simulink model "HVAC_EX"  (Simulink 7.1)
settings: Solver=FixedStepDiscrete  StartTime=0.0  StopTime=40  FixedStep=1  RelTol=1e-3
undefined symbols (not defined in the file or in its folder): AR_A, AR_C, mix_A, mix_C
libraries: MPCMdlLib x21
settings Model: Creator=vichik  LastModifiedBy=vichik

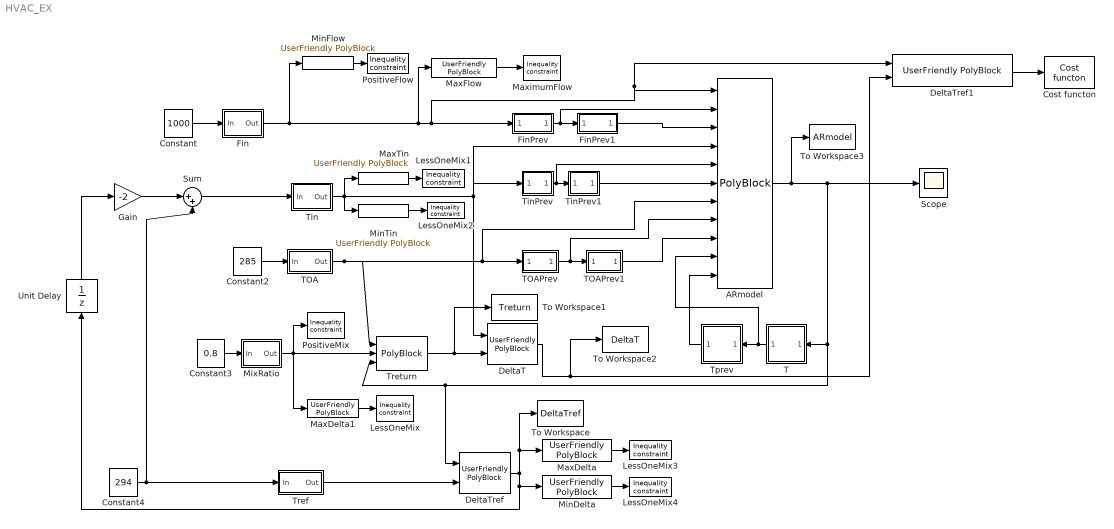
== system HVAC_EX ==
  ARmodel : MPCMdlLib/PolyBlock  Tag=PolyBlock  A=AR_A  C=AR_C
  Constant : Constant  Value=1000  OutDataType=sfix(16)  OutScaling=2^0
  Constant2 : Constant  Value=285  OutDataType=sfix(16)  OutScaling=2^0
  Constant3 : Constant  Value=0.8  OutDataType=sfix(16)  OutScaling=2^0
  Constant4 : Constant  Value=294  OutDataType=sfix(16)  OutScaling=2^0
  Cost functon : MPCMdlLib/Cost functon  Tag=OptCost
  DeltaT : MPCMdlLib/UserFriendly PolyBlock  Tag=PolyBlock  A="[1  0  ; 0 1 ]"  C="[1  -1]"  gA=[0 0]  gC=1
  DeltaTref : MPCMdlLib/UserFriendly PolyBlock  Tag=PolyBlock  A="[1  0  ; 0 1 ]"  C="[1  -1]"  gA=[0 0]  gC=1
  DeltaTref1 : MPCMdlLib/UserFriendly PolyBlock  Tag=PolyBlock  A="[2  0  ; 0 2 ]"  C=[0.00001 1]  gA=[0 0]  gC=1
  Fin : Subsystem  Tag=OptInput  AncestorBlock=MPCMdlLib/Input var  mask{step_ratio=1}
      mask prompts: step_ratio "Step ratio"
      mask Display: fprintf('Input')
  FinPrev : Subsystem  Tag=OptState  AncestorBlock=MPCMdlLib/state  mask{init_val=1000}
      mask prompts: init_val "Initial value"
      mask Display: fprintf('state')
  FinPrev1 : Subsystem  Tag=OptState  AncestorBlock=MPCMdlLib/state  mask{init_val=1000}
      mask prompts: init_val "Initial value"
      mask Display: fprintf('state')
  Gain : Gain  Gain=-2  ParameterDataType=sfix(16)  ParameterScaling=2^0  OutDataType=sfix(16)  OutScaling=2^0
  LessOneMix{,1..4} (5 alike) : MPCMdlLib/Inequality constraint  Tag=InequalBlock  CompareSign=> 0
  MaxDelta : MPCMdlLib/UserFriendly PolyBlock  Tag=PolyBlock  A="[0  ;1]"  C=[2 -1]  gA=[0 ]  gC=1
  MaxDelta1 : MPCMdlLib/UserFriendly PolyBlock  Tag=PolyBlock  A="[0  ;1]"  C=[1 -1]  gA=[0 ]  gC=1
  MaxFlow : MPCMdlLib/UserFriendly PolyBlock  Tag=PolyBlock  A="[0  ; 1]"  C=[4000 -1]  gA=[0 ]  gC=1
  MaxTin : MPCMdlLib/UserFriendly PolyBlock  Tag=PolyBlock  A="[0  ; 1]"  C=[310 -1]  gA=[0 ]  gC=1
  MaximumFlow : MPCMdlLib/Inequality constraint  Tag=InequalBlock  CompareSign=> 0
  MinDelta : MPCMdlLib/UserFriendly PolyBlock  Tag=PolyBlock  A="[1  ; 0]"  C=[1 2]  gA=[0 ]  gC=1
  MinFlow : MPCMdlLib/UserFriendly PolyBlock  Tag=PolyBlock  A="[1  ; 0]"  C=[1 -50]  gA=[0 ]  gC=1
  MinTin : MPCMdlLib/UserFriendly PolyBlock  Tag=PolyBlock  A="[1  ; 0]"  C=[1 -260]  gA=[0 ]  gC=1
  MixRatio : Subsystem  Tag=OptInput  AncestorBlock=MPCMdlLib/Input var  mask{step_ratio=1}
      mask prompts: step_ratio "Step ratio"
      mask Display: fprintf('Input')
  PositiveFlow : MPCMdlLib/Inequality constraint  Tag=InequalBlock  CompareSign=> 0
  PositiveMix : MPCMdlLib/Inequality constraint  Tag=InequalBlock  CompareSign=> 0
  Scope : Scope
      settings: TimeRange=10
  Sum : Sum  Inputs=|++  OutDataType=sfix(16)  OutScaling=2^0
  T : Subsystem  Tag=OptState  Orientation=left  AncestorBlock=MPCMdlLib/state  mask{init_val=293}
      mask prompts: init_val "Initial value"
      mask Display: fprintf('state')
  TOA : Subsystem  Tag=OptExternal  AncestorBlock=MPCMdlLib/External Var
      mask Display: fprintf('External')
  TOAPrev : Subsystem  Tag=OptState  AncestorBlock=MPCMdlLib/state  mask{init_val=285}
      mask prompts: init_val "Initial value"
      mask Display: fprintf('state')
  TOAPrev1 : Subsystem  Tag=OptState  AncestorBlock=MPCMdlLib/state  mask{init_val=285}
      mask prompts: init_val "Initial value"
      mask Display: fprintf('state')
  Tin : Subsystem  Tag=OptInput  AncestorBlock=MPCMdlLib/Input var  mask{step_ratio=1}
      mask prompts: step_ratio "Step ratio"
      mask Display: fprintf('Input')
  TinPrev : Subsystem  Tag=OptState  AncestorBlock=MPCMdlLib/state  mask{init_val=294}
      mask prompts: init_val "Initial value"
      mask Display: fprintf('state')
  TinPrev1 : Subsystem  Tag=OptState  AncestorBlock=MPCMdlLib/state  mask{init_val=294}
      mask prompts: init_val "Initial value"
      mask Display: fprintf('state')
  To Workspace : ToWorkspace  VariableName=DeltaTref  SampleTime=-1  SaveFormat=Structure
  To Workspace1 : ToWorkspace  VariableName=Treturn  SampleTime=-1  SaveFormat=Structure
  To Workspace2 : ToWorkspace  VariableName=DeltaT  SampleTime=-1  SaveFormat=Structure
  To Workspace3 : ToWorkspace  VariableName=ARmodel  SampleTime=-1  SaveFormat=Structure With Time
  Tprev : Subsystem  Tag=OptState  Orientation=left  AncestorBlock=MPCMdlLib/state  mask{init_val=293}
      mask prompts: init_val "Initial value"
      mask Display: fprintf('state')
  Tref : Subsystem  Tag=OptExternal  AncestorBlock=MPCMdlLib/External Var
      mask Display: fprintf('External')
  Treturn : MPCMdlLib/PolyBlock  Tag=PolyBlock  A=mix_A  C=mix_C
  Unit Delay : UnitDelay  Orientation=up  SampleTime=-1
  wires:
  Constant/1 -> Fin/1(In)
  Fin/1(Out) -> FinPrev/1(In1), ARmodel/1, DeltaTref1/1, MaxFlow/1, MinFlow/1
  Tin/1(Out) -> TinPrev/1(In1), DeltaT/1, ARmodel/4, MinTin/1, MaxTin/1
  FinPrev/1(Out1) -> FinPrev1/1(In1), ARmodel/2
  Constant2/1 -> TOA/1(In)
  TOA/1(Out) -> Treturn/1, TOAPrev/1(In1), ARmodel/7
  MaxFlow/1 -> MaximumFlow/1
  Constant3/1 -> MixRatio/1(In)
  MixRatio/1(Out) -> PositiveMix/1, MaxDelta1/1, Treturn/2
  MaxDelta1/1 -> LessOneMix/1
  MaxTin/1 -> LessOneMix1/1
  MinTin/1 -> LessOneMix2/1
  T/1(Out1) -> Tprev/1(In1), ARmodel/10
  ARmodel/1 -> T/1(In1), DeltaTref/1, Treturn/3, Scope/1, To Workspace3/1
  Treturn/1 -> To Workspace1/1, DeltaT/2
  Constant4/1 -> Tref/1(In), Sum/2
  Tref/1(Out) -> DeltaTref/2
  DeltaTref/1 -> Unit Delay/1, MinDelta/1, To Workspace/1, MaxDelta/1
  DeltaT/1 -> To Workspace2/1, DeltaTref1/2
  DeltaTref1/1 -> Cost functon/1
  TinPrev/1(Out1) -> TinPrev1/1(In1), ARmodel/5
  FinPrev1/1(Out1) -> ARmodel/3
  TinPrev1/1(Out1) -> ARmodel/6
  TOAPrev/1(Out1) -> TOAPrev1/1(In1), ARmodel/8
  TOAPrev1/1(Out1) -> ARmodel/9
  Tprev/1(Out1) -> ARmodel/11
  Sum/1 -> Tin/1(In)
  Gain/1 -> Sum/1
  Unit Delay/1 -> Gain/1
  MinFlow/1 -> PositiveFlow/1
  MinDelta/1 -> LessOneMix4/1
  MaxDelta/1 -> LessOneMix3/1

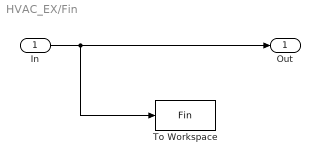
== system HVAC_EX/Fin ==
  In : Inport  OutDataType=fixdt(1, 16)  OutScaling=2^0
  To Workspace : ToWorkspace  VariableName=Fin  SampleTime=-1  SaveFormat=Structure
      settings: InitFcn=set_param(getfullname(gcb),'VariableName',get_param(get_param(gcb,'parent'),'name'))
  Out : Outport  OutDataType=fixdt(1, 16)  OutScaling=2^0
  wires:
  In/1 -> To Workspace/1, Out/1

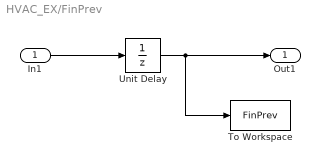
== system HVAC_EX/FinPrev ==
  In1 : Inport  OutDataType=fixdt(1, 16)  OutScaling=2^0
  To Workspace : ToWorkspace  VariableName=FinPrev  SampleTime=-1  SaveFormat=Structure
      settings: InitFcn=set_param(getfullname(gcb),'VariableName',get_param(get_param(gcb,'parent'),'name'))
  Unit Delay : UnitDelay  X0=init_val  SampleTime=-1
  Out1 : Outport  OutDataType=fixdt(1, 16)  OutScaling=2^0
  wires:
  Unit Delay/1 -> To Workspace/1, Out1/1
  In1/1 -> Unit Delay/1

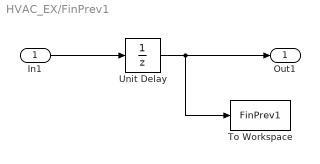
== system HVAC_EX/FinPrev1 ==
  In1 : Inport  OutDataType=fixdt(1, 16)  OutScaling=2^0
  To Workspace : ToWorkspace  VariableName=FinPrev1  SampleTime=-1  SaveFormat=Structure
      settings: InitFcn=set_param(getfullname(gcb),'VariableName',get_param(get_param(gcb,'parent'),'name'))
  Unit Delay : UnitDelay  X0=init_val  SampleTime=-1
  Out1 : Outport  OutDataType=fixdt(1, 16)  OutScaling=2^0
  wires:
  Unit Delay/1 -> To Workspace/1, Out1/1
  In1/1 -> Unit Delay/1

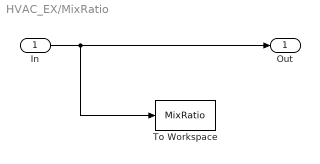
== system HVAC_EX/MixRatio ==
  In : Inport  OutDataType=fixdt(1, 16)  OutScaling=2^0
  To Workspace : ToWorkspace  VariableName=MixRatio  SampleTime=-1  SaveFormat=Structure
      settings: InitFcn=set_param(getfullname(gcb),'VariableName',get_param(get_param(gcb,'parent'),'name'))
  Out : Outport  OutDataType=fixdt(1, 16)  OutScaling=2^0
  wires:
  In/1 -> To Workspace/1, Out/1

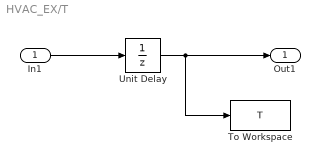
== system HVAC_EX/T ==
  In1 : Inport  OutDataType=fixdt(1, 16)  OutScaling=2^0
  To Workspace : ToWorkspace  VariableName=T  SampleTime=-1  SaveFormat=Structure
      settings: InitFcn=set_param(getfullname(gcb),'VariableName',get_param(get_param(gcb,'parent'),'name'))
  Unit Delay : UnitDelay  X0=init_val  SampleTime=-1
  Out1 : Outport  OutDataType=fixdt(1, 16)  OutScaling=2^0
  wires:
  Unit Delay/1 -> To Workspace/1, Out1/1
  In1/1 -> Unit Delay/1

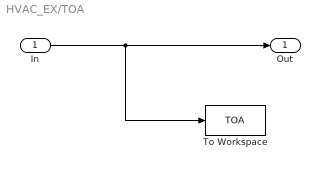
== system HVAC_EX/TOA ==
  In : Inport  OutDataType=fixdt(1, 16)  OutScaling=2^0
  To Workspace : ToWorkspace  VariableName=TOA  SampleTime=-1  SaveFormat=Structure
      settings: InitFcn=set_param(getfullname(gcb),'VariableName',get_param(get_param(gcb,'parent'),'name'))
  Out : Outport  OutDataType=fixdt(1, 16)  OutScaling=2^0
  wires:
  In/1 -> To Workspace/1, Out/1

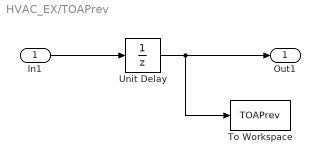
== system HVAC_EX/TOAPrev ==
  In1 : Inport  OutDataType=fixdt(1, 16)  OutScaling=2^0
  To Workspace : ToWorkspace  VariableName=TOAPrev  SampleTime=-1  SaveFormat=Structure
      settings: InitFcn=set_param(getfullname(gcb),'VariableName',get_param(get_param(gcb,'parent'),'name'))
  Unit Delay : UnitDelay  X0=init_val  SampleTime=-1
  Out1 : Outport  OutDataType=fixdt(1, 16)  OutScaling=2^0
  wires:
  Unit Delay/1 -> To Workspace/1, Out1/1
  In1/1 -> Unit Delay/1

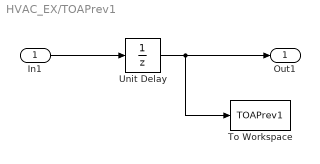
== system HVAC_EX/TOAPrev1 ==
  In1 : Inport  OutDataType=fixdt(1, 16)  OutScaling=2^0
  To Workspace : ToWorkspace  VariableName=TOAPrev1  SampleTime=-1  SaveFormat=Structure
      settings: InitFcn=set_param(getfullname(gcb),'VariableName',get_param(get_param(gcb,'parent'),'name'))
  Unit Delay : UnitDelay  X0=init_val  SampleTime=-1
  Out1 : Outport  OutDataType=fixdt(1, 16)  OutScaling=2^0
  wires:
  Unit Delay/1 -> To Workspace/1, Out1/1
  In1/1 -> Unit Delay/1

== system HVAC_EX/Tin ==
  In : Inport  OutDataType=fixdt(1, 16)  OutScaling=2^0
  To Workspace : ToWorkspace  VariableName=Tin  SampleTime=-1  SaveFormat=Structure
      settings: InitFcn=set_param(getfullname(gcb),'VariableName',get_param(get_param(gcb,'parent'),'name'))
  Out : Outport  OutDataType=fixdt(1, 16)  OutScaling=2^0
  wires:
  In/1 -> To Workspace/1, Out/1

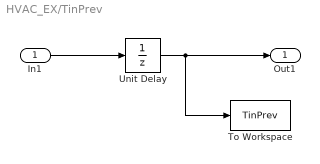
== system HVAC_EX/TinPrev ==
  In1 : Inport  OutDataType=fixdt(1, 16)  OutScaling=2^0
  To Workspace : ToWorkspace  VariableName=TinPrev  SampleTime=-1  SaveFormat=Structure
      settings: InitFcn=set_param(getfullname(gcb),'VariableName',get_param(get_param(gcb,'parent'),'name'))
  Unit Delay : UnitDelay  X0=init_val  SampleTime=-1
  Out1 : Outport  OutDataType=fixdt(1, 16)  OutScaling=2^0
  wires:
  Unit Delay/1 -> To Workspace/1, Out1/1
  In1/1 -> Unit Delay/1

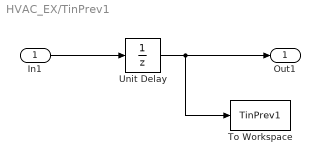
== system HVAC_EX/TinPrev1 ==
  In1 : Inport  OutDataType=fixdt(1, 16)  OutScaling=2^0
  To Workspace : ToWorkspace  VariableName=TinPrev1  SampleTime=-1  SaveFormat=Structure
      settings: InitFcn=set_param(getfullname(gcb),'VariableName',get_param(get_param(gcb,'parent'),'name'))
  Unit Delay : UnitDelay  X0=init_val  SampleTime=-1
  Out1 : Outport  OutDataType=fixdt(1, 16)  OutScaling=2^0
  wires:
  Unit Delay/1 -> To Workspace/1, Out1/1
  In1/1 -> Unit Delay/1

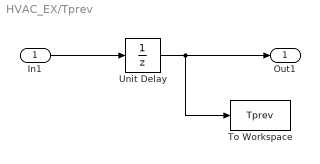
== system HVAC_EX/Tprev ==
  In1 : Inport  OutDataType=fixdt(1, 16)  OutScaling=2^0
  To Workspace : ToWorkspace  VariableName=Tprev  SampleTime=-1  SaveFormat=Structure
      settings: InitFcn=set_param(getfullname(gcb),'VariableName',get_param(get_param(gcb,'parent'),'name'))
  Unit Delay : UnitDelay  X0=init_val  SampleTime=-1
  Out1 : Outport  OutDataType=fixdt(1, 16)  OutScaling=2^0
  wires:
  Unit Delay/1 -> To Workspace/1, Out1/1
  In1/1 -> Unit Delay/1

== system HVAC_EX/Tref ==
  In : Inport  OutDataType=fixdt(1, 16)  OutScaling=2^0
  To Workspace : ToWorkspace  VariableName=Tref  SampleTime=-1  SaveFormat=Structure
      settings: InitFcn=set_param(getfullname(gcb),'VariableName',get_param(get_param(gcb,'parent'),'name'))
  Out : Outport  OutDataType=fixdt(1, 16)  OutScaling=2^0
  wires:
  In/1 -> To Workspace/1, Out/1
